simulink model "sampleModel1475_1"  (R2023a)
settings: Solver=VariableStepAuto  StartTime=0.0  StopTime=10.0  RelTol=1e-3
libraries: hdlsllib x3
settings Model: Creator=user1  LastModifiedBy=user1

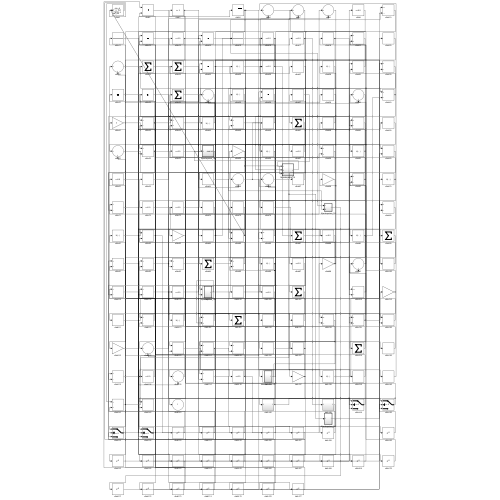
[thumbnail: Simulink's stored preview of the top-level diagram]
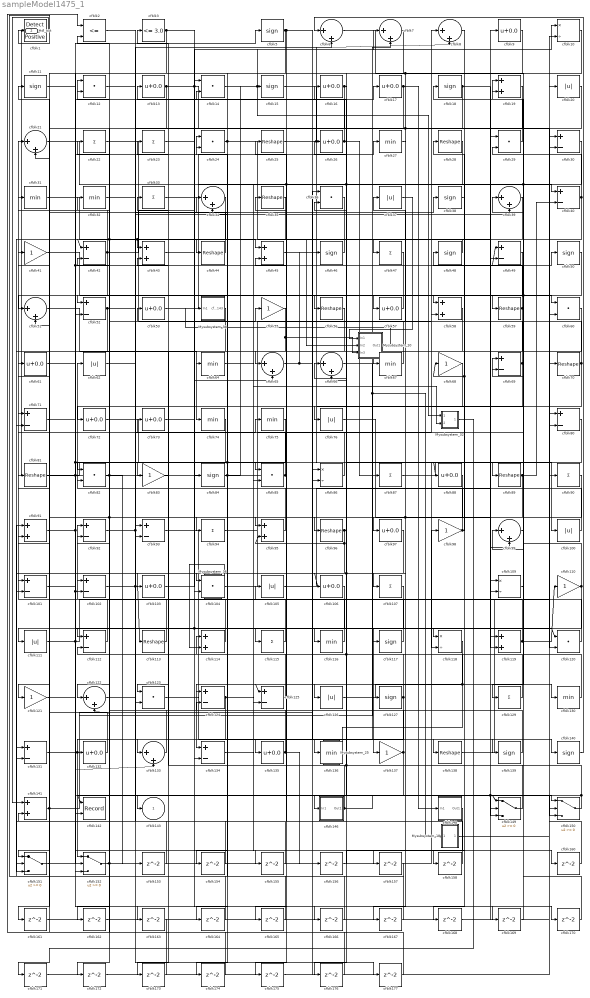
== system sampleModel1475_1 ==
  Mysubsystem_10 : Subsystem  TreatAsAtomicUnit=on  RTWFcnName=Mysubsystem_10
      settings: RTWFcnNameOpts=User specified  RTWFileNameOpts=Use function name
  Mysubsystem_18 : Subsystem  TreatAsAtomicUnit=on  RTWFcnName=Mysubsystem_18
      settings: RTWFcnNameOpts=User specified  RTWFileNameOpts=Use function name
  Mysubsystem_25 : Subsystem  TreatAsAtomicUnit=on  RTWFcnName=Mysubsystem_25
      settings: RTWFcnNameOpts=User specified  RTWFileNameOpts=Use function name
  Mysubsystem_32 : Subsystem  TreatAsAtomicUnit=on  RTWFcnName=Mysubsystem_32
      settings: RTWFcnNameOpts=User specified  RTWFileNameOpts=Use function name
  Mysubsystem_36 : Subsystem  TreatAsAtomicUnit=on  RTWFcnName=Mysubsystem_36
      settings: RTWFcnNameOpts=User specified  RTWFileNameOpts=Use function name
  Mysubsystem_38 : Subsystem  TreatAsAtomicUnit=on  RTWFcnName=Mysubsystem_38
      settings: RTWFcnNameOpts=User specified  RTWFileNameOpts=Use function name
  cfblk1 : hdlsllib/Logic and Bit Operations/Detect Rise Positive  vinit=0  OutDataTypeStr=uint8
  cfblk{10,86,109,118} (4 alike) : Product  Inputs=*/  OutDataTypeStr=uint8  RndMeth=Zero  SaturateOnIntegerOverflow=on
  cfblk{20,37,62,76,100,105,111,126} (8 alike) : Abs  OutDataTypeStr=uint8  SaturateOnIntegerOverflow=off
  cfblk{30,40,42,49,52,69,71,80,92..93,101..102,112,124..125,131,134} (17 alike) : Sum  Inputs=+-  OutDataTypeStr=uint8
  cfblk{9,13,16..17,26,53,57,61,72..73,88,97,103,106,132,135} (16 alike) : Bias  Bias=0.0  SaturateOnIntegerOverflow=off
  cfblk{12,14,24,29,36,60,82,85,104,120,123} (11 alike) : DotProduct  OutDataTypeStr=uint8
  cfblk{22..23,33,47,87,90,94,107,115,129} (10 alike) : Sum  Inputs=+  OutDataTypeStr=uint8
  cfblk{5,11,15,18,38,46,48,50,84,117,127,139..140} (13 alike) : Signum
  cfblk{41,55,68,83,98,110,121,137} (8 alike) : Gain  OutDataTypeStr=uint8
  cfblk{25,28,35,44,56,59,70,81,89,96,113,138} (12 alike) : Reshape
  cfblk{19,43,45,58,91,95,114,119,141} (9 alike) : Sum  OutDataTypeStr=uint8
  cfblk{27,31..32,64,67,74..75,116,130,136} (10 alike) : MinMax  OutDataTypeStr=uint8
  cfblk{6..8,21,34,39,51,65..66,99,122,133} (12 alike) : Sum  Inputs=|++  OutDataTypeStr=uint8
  cfblk142 : Record  FileSettingsInternal="{\"entries\":[{\"content\":{\"excelSettings\":{\"content\":{},\"type\":\"Streamout.ExcelSettings\"}},\"type\":\"Streamout.FileSettingStorage\",\"uuid\":\"\"}],\"packageUris\":[\"http:\\/\\/schema.mathworks.com\\/mf0\\/streamout_blocks\\/R2020a\"],\"version\":\"1.0\"}"  Layout=[1 1]  SignalsInternal="{\"entries\":[{\"content\":{\"signals\":[{\"content\":{\"blockPath\":[],\"dimensions\":[1],\"domain\":\"\",\"lineColor\":\"#a2142f\",\"plots\":[1],\"port\":1,\"signalID\":20115,\"signalName\":\"cfblk150\"},\"type\":\"RecordBlkView.Signal\",\"uuid\":\"\"},{\"content\":{\"blockPath\":[],\"dimensions\":[1],\"domain\":\"\",\"lineColor\":\"#139fff\",\"plots\":[1],\"port\":2,\"signalID\":20118,\"signalName\":\"cfblk75\"},\"type\":\"RecordBlkView.Signal\",\"uuid\":\"\"}]},\"type\":\"RecordBlkView.InputSignals\",\"uuid\":\"\"}],\"packageUris\":[\"http:\\/\\/schema.mathworks.com\\/mf0\\/streamout_blocks\\/R2020a\"],\"version\":\"1.0\"}"  VisualizationBindings="{\"xyplotplugin\":{\"info\":[{\"series\":[{\"bindingParametersList\":[{\"parameter\":\"X-Axis\",\"signalID\":20115,\"signalName\":\"cfblk150\"},{\"parameter\":\"Y-Axis\",\"signalID\":20118,\"signalName\":\"cfblk75\"}],\"seriesID\":16642}],\"subplotID\":1}]}}"  CompatibilityTag=XY  st=-1
  cfblk146 : Subsystem
      settings: LibrarySourceBlock=|
      | hdlsllib/Ports &
      | Subsystems/Subsystem
  cfblk148 : Subsystem
      settings: LibrarySourceBlock=|
      | hdlsllib/Ports &
      | Subsystems/Subsystem
  cfblk{149..152} (4 alike) : Switch  OutDataTypeStr=uint8  SaturateOnIntegerOverflow=off  InputSameDT=off
  cfblk{153..158,160..177} (24 alike) : Delay  SampleTime=1
  cfblk2 : RelationalOperator  Operator=<=  OutDataTypeStr=boolean  InputSameDT=off
  cfblk3 : hdlsllib/Logic and Bit Operations/Compare To Constant  relop=<=  const=3.0  OutDataTypeStr=uint8
  cfblk143 : Outport  OutDataTypeStr=uint8  VectorParamsAs1DForOutWhenUnconnected=off
  Hdl_out : Outport  Port=2  OutDataTypeStr=uint8
  wires:
  cfblk115/1 -> cfblk92/1
  cfblk48/1 -> cfblk47/1
  cfblk14/1 -> Mysubsystem_32/1(In1), cfblk7/1
  cfblk66/1 -> Mysubsystem_18/1(In1), cfblk140/1
  cfblk73/1 -> cfblk120/1, cfblk157/1
  cfblk17/1 -> cfblk148/1(In1), cfblk175/1
  cfblk124/1 -> cfblk149/1, cfblk149/3, cfblk152/1
  cfblk65/1 -> cfblk86/2, cfblk46/1
  cfblk53/1 -> cfblk27/1
  cfblk97/1 -> cfblk131/2
  cfblk118/1 -> cfblk134/1
  cfblk6/1 -> cfblk118/1
  cfblk22/1 -> cfblk55/1
  cfblk125/1 -> cfblk23/1
  cfblk100/1 -> cfblk62/1
  cfblk85/1 -> cfblk13/1, Hdl_out/1
  cfblk18/1 -> cfblk124/1, cfblk127/1, cfblk109/1
  cfblk119/1 -> cfblk110/1, cfblk25/1
  cfblk87/1 -> cfblk89/1
  cfblk96/1 -> cfblk95/2, cfblk154/1, cfblk146/1(In1)
  cfblk59/1 -> cfblk123/1, cfblk28/1
  cfblk3/1 -> cfblk152/3, cfblk169/1
  cfblk81/1 -> cfblk83/1, cfblk166/1
  cfblk55/1 -> Mysubsystem_10/3(In3), cfblk71/2
  cfblk31/1 -> cfblk45/1
  cfblk1/1 -> cfblk141/1
  cfblk140/1 -> cfblk6/1
  cfblk107/1 -> cfblk111/1
  cfblk10/1 -> cfblk67/1, cfblk76/1
  cfblk91/1 -> cfblk50/1, cfblk133/2
  cfblk33/1 -> cfblk40/1
  cfblk9/1 -> cfblk97/1
  cfblk72/1 -> cfblk100/1
  cfblk29/1 -> cfblk18/1
  cfblk109/1 -> cfblk39/1
  cfblk42/1 -> cfblk21/1, cfblk17/1, cfblk152/2
  cfblk104/1 -> cfblk8/1
  cfblk138/1 -> cfblk70/1
  cfblk74/1 -> cfblk93/2
  cfblk93/1 -> cfblk139/1
  cfblk30/1 -> cfblk85/1, cfblk85/2, cfblk59/1
  cfblk132/1 -> cfblk11/1
  cfblk16/1 -> cfblk126/1, cfblk106/1, cfblk94/1
  cfblk44/1 -> cfblk21/2
  cfblk61/1 -> cfblk5/1, cfblk49/1
  cfblk68/1 -> cfblk122/1
  cfblk95/1 -> cfblk32/1
  cfblk106/1 -> cfblk134/2
  cfblk113/1 -> cfblk31/1
  cfblk67/1 -> cfblk53/1
  cfblk110/1 -> cfblk137/1, cfblk71/1
  cfblk47/1 -> cfblk151/1
  cfblk15/1 -> cfblk118/2
  cfblk20/1 -> cfblk72/1
  cfblk92/1 -> cfblk75/1, cfblk116/1
  cfblk41/1 -> cfblk60/1
  cfblk135/1 -> cfblk34/1, cfblk156/1
  cfblk98/1 -> cfblk48/1, cfblk68/1, cfblk66/2
  cfblk62/1 -> cfblk39/2
  cfblk122/1 -> cfblk38/1
  cfblk131/1 -> cfblk36/1, cfblk132/1
  cfblk51/1 -> cfblk74/1
  cfblk69/1 -> cfblk12/1, cfblk103/1
  cfblk149/1 -> cfblk33/1, cfblk16/1
  cfblk139/1 -> cfblk102/1
  cfblk84/1 -> cfblk24/1, cfblk15/1
  cfblk46/1 -> cfblk44/1
  cfblk90/1 -> cfblk121/1, cfblk162/1
  cfblk70/1 -> cfblk37/1, cfblk120/2
  cfblk50/1 -> cfblk125/2, cfblk129/1
  cfblk126/1 -> cfblk130/1
  cfblk49/1 -> cfblk65/1
  cfblk5/1 -> cfblk95/1, cfblk138/1, cfblk51/1
  cfblk123/1 -> cfblk135/1
  cfblk105/1 -> cfblk9/1
  cfblk27/1 -> cfblk57/1
  cfblk11/1 -> cfblk102/2, cfblk150/3
  cfblk24/1 -> cfblk109/2, cfblk164/1
  cfblk111/1 -> cfblk20/1, cfblk14/2, cfblk170/1
  cfblk25/1 -> cfblk8/2, cfblk49/2
  cfblk99/1 -> cfblk29/2
  cfblk133/1 -> cfblk101/1
  cfblk34/1 -> cfblk101/2
  cfblk13/1 -> cfblk90/1, cfblk10/1, cfblk161/1
  cfblk141/1 -> cfblk91/2, cfblk7/2
  cfblk150/1 -> cfblk114/1, cfblk142/1
  cfblk45/1 -> cfblk80/2
  cfblk130/1 -> cfblk19/1
  cfblk56/1 -> cfblk123/2
  cfblk7/1 -> cfblk64/1
  cfblk83/1 -> cfblk133/1
  cfblk21/1 -> cfblk84/1
  cfblk129/1 -> cfblk34/2
  cfblk32/1 -> cfblk56/1
  cfblk152/1 -> cfblk98/1, cfblk22/1
  cfblk80/1 -> cfblk96/1
  cfblk146/1(Out1) -> cfblk73/1, cfblk149/2
  cfblk35/1 -> cfblk42/1, cfblk122/2
  cfblk43/1 -> cfblk65/2
  cfblk26/1 -> cfblk3/1, cfblk87/1
  cfblk89/1 -> cfblk107/1, cfblk172/1, cfblk40/2
  cfblk60/1 -> cfblk119/2
  cfblk151/1 -> cfblk24/2
  cfblk57/1 -> cfblk52/1
  cfblk112/1 -> cfblk61/1
  cfblk102/1 -> cfblk113/1, cfblk177/1
  cfblk117/1 -> cfblk105/1
  cfblk103/1 -> cfblk14/1
  cfblk127/1 -> cfblk92/2, cfblk26/1, cfblk173/1
  cfblk82/1 -> cfblk112/1, cfblk153/1
  cfblk76/1 -> cfblk99/2
  cfblk136/1 -> cfblk66/1
  cfblk52/1 -> cfblk6/2, cfblk151/3
  cfblk116/1 -> cfblk81/1
  cfblk38/1 -> cfblk58/1
  cfblk36/1 -> cfblk82/1, cfblk43/1
  cfblk94/1 -> cfblk58/2
  cfblk2/1 -> cfblk30/2
  cfblk12/1 -> cfblk150/1
  cfblk75/1 -> cfblk104/1, cfblk142/2
  cfblk71/1 -> cfblk115/1, cfblk88/1
  cfblk86/1 -> cfblk35/1
  cfblk137/1 -> cfblk2/2, cfblk174/1
  cfblk40/1 -> cfblk52/2, cfblk19/2
  cfblk114/1 -> cfblk41/1
  cfblk28/1 -> cfblk104/2, cfblk136/1
  cfblk23/1 -> cfblk117/1
  cfblk120/1 -> cfblk69/1
  cfblk153/1 -> cfblk141/2
  cfblk154/1 -> cfblk93/1
  cfblk101/1 -> cfblk155/1
  cfblk155/1 -> cfblk91/1
  cfblk156/1 -> cfblk36/2
  cfblk157/1 -> cfblk1/1
  cfblk8/1 -> cfblk158/1
  cfblk158/1 -> cfblk45/2
  cfblk134/1 -> cfblk160/1
  cfblk160/1 -> cfblk150/2
  cfblk161/1 -> cfblk119/1
  cfblk162/1 -> cfblk60/2
  cfblk121/1 -> cfblk163/1
  cfblk163/1 -> cfblk2/1
  cfblk164/1 -> cfblk151/2
  cfblk58/1 -> cfblk165/1
  cfblk165/1 -> cfblk131/1
  cfblk166/1 -> cfblk124/2
  cfblk88/1 -> cfblk167/1
  cfblk167/1 -> cfblk12/2
  cfblk19/1 -> cfblk168/1
  cfblk168/1 -> cfblk29/1
  cfblk169/1 -> cfblk99/1
  cfblk170/1 -> cfblk69/2
  cfblk171/1 -> cfblk80/1
  cfblk172/1 -> cfblk10/2
  cfblk173/1 -> cfblk112/2
  cfblk174/1 -> cfblk82/2
  cfblk175/1 -> cfblk86/1
  cfblk148/1(Out1) -> cfblk176/1
  cfblk176/1 -> cfblk42/2
  cfblk177/1 -> cfblk51/2
  cfblk37/1 -> Mysubsystem_10/1(In1)
  cfblk39/1 -> Mysubsystem_10/2(In2)
  Mysubsystem_18/1(Out1) -> cfblk30/1
  Mysubsystem_25/1(Out1) -> cfblk125/1, cfblk43/2
  cfblk64/1 -> Mysubsystem_32/2(In2)
  Mysubsystem_32/1(Out1) -> cfblk171/1
  Mysubsystem_36/1(Out1) -> cfblk114/2
  Mysubsystem_10/1(Out1) -> Mysubsystem_38/1(In1)
  Mysubsystem_38/1(cfblk143) -> cfblk143/1

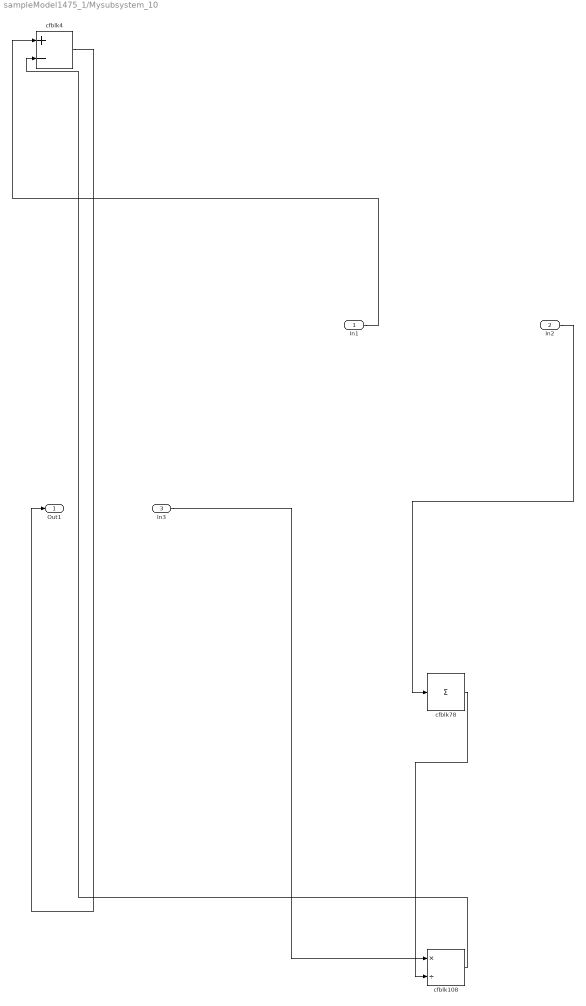
== system sampleModel1475_1/Mysubsystem_10 ==
  In1 : Inport
  In2 : Inport  Port=2
  In3 : Inport  Port=3
  cfblk108 : Product  Inputs=*/  RndMeth=Zero  SaturateOnIntegerOverflow=on
  cfblk4 : Sum  Inputs=+-
  cfblk78 : Sum  Inputs=+
  Out1 : Outport
  wires:
  cfblk78/1 -> cfblk108/2
  cfblk108/1 -> cfblk4/2
  In2/1 -> cfblk78/1
  In1/1 -> cfblk4/1
  cfblk4/1 -> Out1/1
  In3/1 -> cfblk108/1

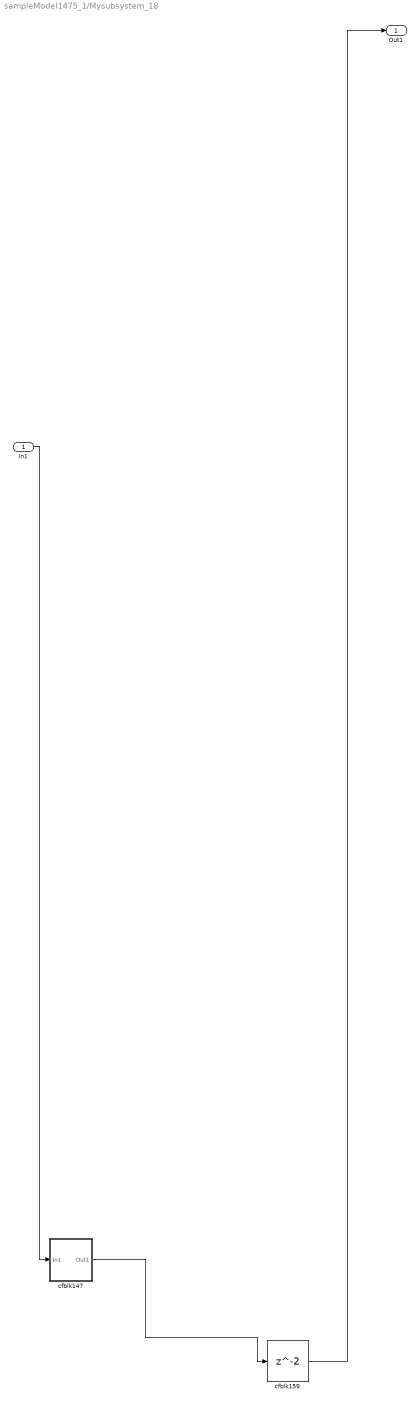
== system sampleModel1475_1/Mysubsystem_18 ==
  In1 : Inport
  cfblk147 : Subsystem
      settings: LibrarySourceBlock=|
      | hdlsllib/Ports &
      | Subsystems/Subsystem
  cfblk159 : Delay  SampleTime=1
  Out1 : Outport
  wires:
  cfblk147/1(Out1) -> cfblk159/1
  In1/1 -> cfblk147/1(In1)
  cfblk159/1 -> Out1/1

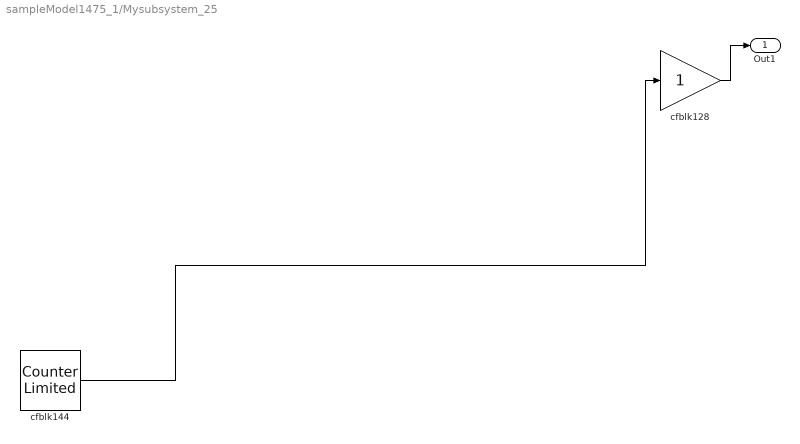
== system sampleModel1475_1/Mysubsystem_25 ==
  cfblk128 : Gain
  cfblk144 : hdlsllib/Sources/Counter Limited  uplimit=7  tsamp=-1
  Out1 : Outport
  wires:
  cfblk144/1 -> cfblk128/1
  cfblk128/1 -> Out1/1

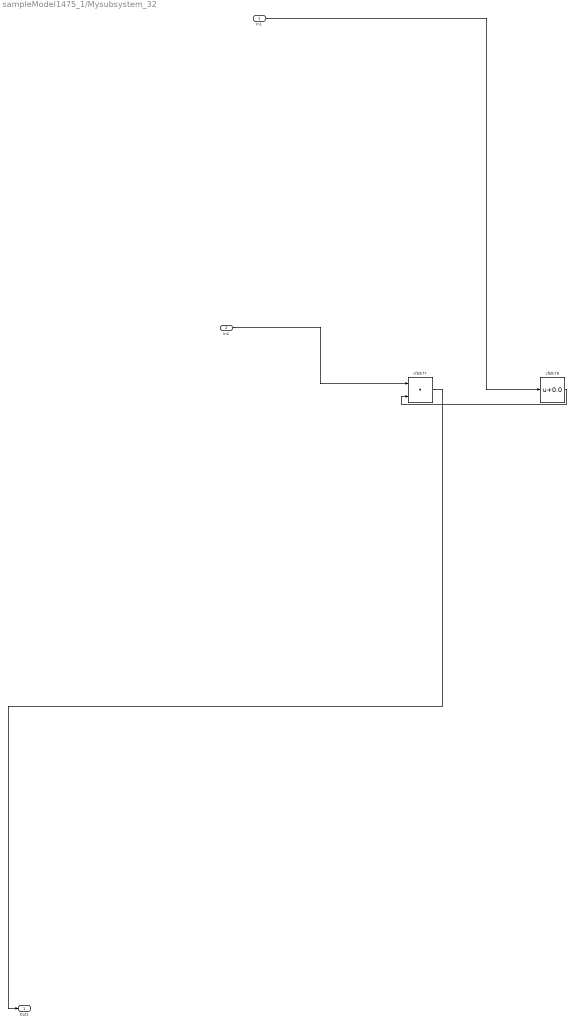
== system sampleModel1475_1/Mysubsystem_32 ==
  In1 : Inport
  In2 : Inport  Port=2
  cfblk77 : DotProduct  OutDataTypeStr=Inherit: Inherit via internal rule
  cfblk79 : Bias  Bias=0.0  SaturateOnIntegerOverflow=off
  Out1 : Outport
  wires:
  cfblk79/1 -> cfblk77/2
  In1/1 -> cfblk79/1
  cfblk77/1 -> Out1/1
  In2/1 -> cfblk77/1

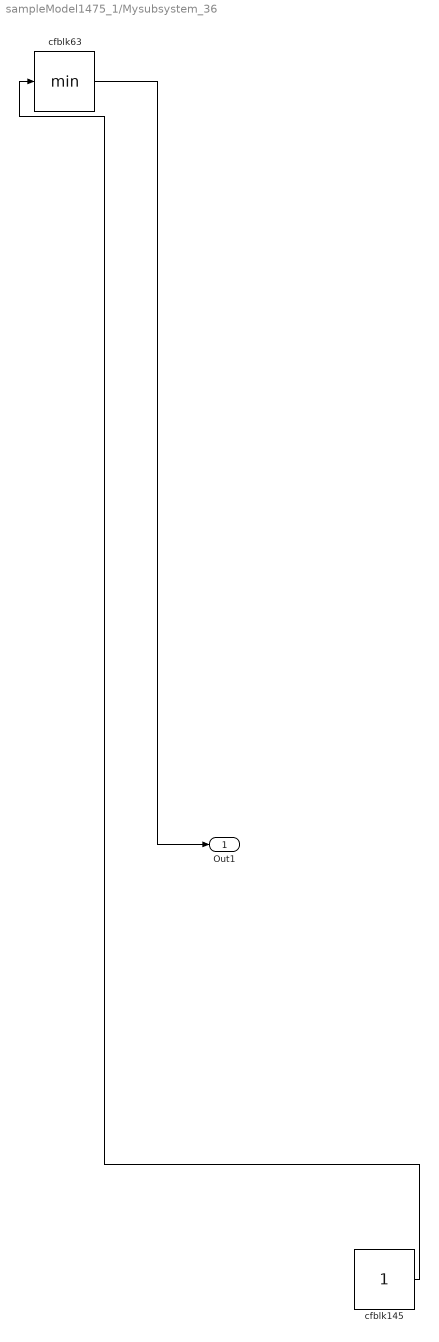
== system sampleModel1475_1/Mysubsystem_36 ==
  cfblk145 : Constant  SampleTime=-1
  cfblk63 : MinMax
  Out1 : Outport
  wires:
  cfblk145/1 -> cfblk63/1
  cfblk63/1 -> Out1/1

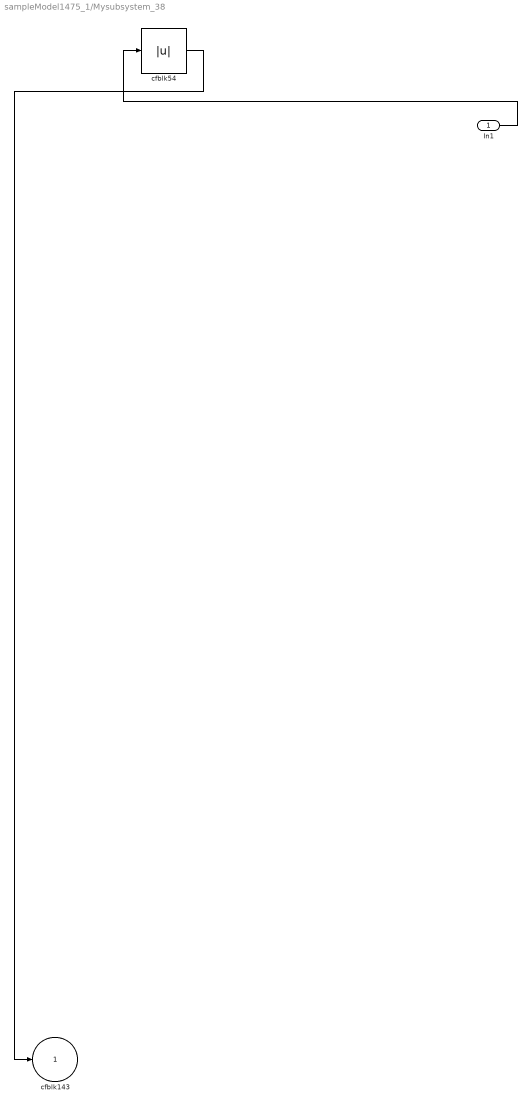
== system sampleModel1475_1/Mysubsystem_38 ==
  In1 : Inport
  cfblk54 : Abs  SaturateOnIntegerOverflow=off
  cfblk143 : Outport  VectorParamsAs1DForOutWhenUnconnected=off
  wires:
  cfblk54/1 -> cfblk143/1
  In1/1 -> cfblk54/1

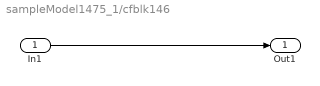
== system sampleModel1475_1/cfblk146 ==
  In1 : Inport
  Out1 : Outport
  wires:
  In1/1 -> Out1/1

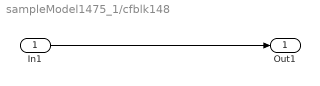
== system sampleModel1475_1/cfblk148 ==
  In1 : Inport
  Out1 : Outport
  wires:
  In1/1 -> Out1/1

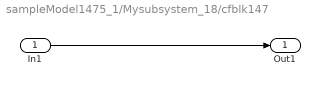
== system sampleModel1475_1/Mysubsystem_18/cfblk147 ==
  In1 : Inport
  Out1 : Outport
  wires:
  In1/1 -> Out1/1
